simulink model "Assignment"  (Simulink 7.3)
settings: Solver=ode45  StartTime=0.0  StopTime=150  RelTol=1e-3
libraries: simulink_extras x1
settings Model: Creator=Ben  LastModifiedBy=Ben

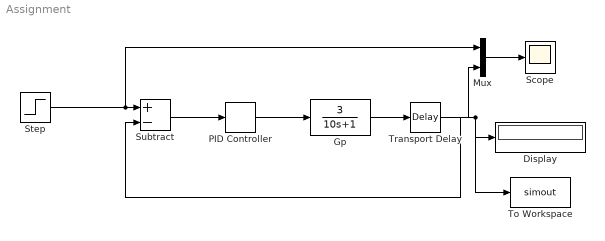
== system Assignment ==
  Display : Display
  Gp : TransferFcn  Numerator=[3]  Denominator=[10 1]
  Mux : Mux  Inputs=2
  PID Controller : simulink_extras/Additional Linear/PID Controller  SystemSampleTime=-1  P=0.2  I=0.09  D=0
  Scope : Scope
  Step : Step  SampleTime=4
  Subtract : Sum  Inputs=+-  OutDataType=fixdt(1, 16)  OutScaling=2^-10
  To Workspace : ToWorkspace  VariableName=simout  SampleTime=-1  SaveFormat=Structure
  Transport Delay : TransportDelay  DelayTime=2  InitialOutput=2
  wires:
  Gp/1 -> Transport Delay/1
  Subtract/1 -> PID Controller/1
  PID Controller/1 -> Gp/1
  Transport Delay/1 -> To Workspace/1, Subtract/2, Display/1, Mux/2
  Step/1 -> Subtract/1, Mux/1
  Mux/1 -> Scope/1
